simulink model "Bruss"  (Simulink 7.9)
settings: Solver=ode45  StartTime=0.0  StopTime=10.0  RelTol=1e-3
libraries: simulink x1
settings Model: Creator=Yi  LastModifiedBy=parasara

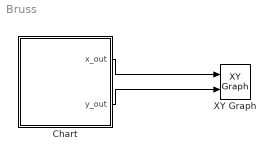
== system Bruss ==
  Chart : Stateflow chart  TreatAsAtomicUnit=on
  XY Graph : simulink/Sinks/XY Graph  xmin=0  xmax=5  ymin=0  ymax=5  st=-1
  wires:
  Chart/1(x_out) -> XY Graph/1
  Chart/2(y_out) -> XY Graph/2

== stateflow chart Chart ==
  settings: updateMethod=CONTINUOUS
  state Brussellator
    du:
    x_dot = 1 + x*x*y - 2.5*x;
    y_dot = 1.5*x - x*x*y;
    x_out = x;
    y_out = y;
  note: @annotation-mode=Brussellator;
      | k=2000.0;
      | gamma=0.0;
  (default) -> Brussellator : {x=0.95, y=0.05}
  data: x local double; y local double; x_out output double; y_out output double
  data x settings: updateMethod=SF_CONTINUOUS_TIME_DATA
  data y settings: updateMethod=SF_CONTINUOUS_TIME_DATA
